simulink model "untitled"  (R2021a)
settings: Solver=VariableStepAuto  StartTime=0.0  StopTime=10.0  RelTol=1e-3
settings Model: Creator=nguye  LastModifiedBy=nguye

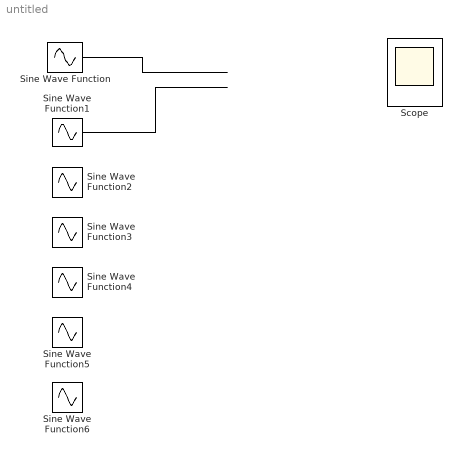
== system untitled ==
  Scope : Scope
  Sine Wave Function : Sin  Amplitude=2  Frequency=30  Phase=pi/2  SampleTime=1/10000
  Sine Wave Function1 : Sin  Amplitude=0.08  Frequency=30  Phase=0.05*pi  SampleTime=1/10000
  Sine Wave Function{2..6} (5 alike) : Sin  TimeSource=Use external signal  SampleTime=0
  wires:
  Sine Wave Function/1 -> ?
  Sine Wave Function1/1 -> ?
  ? -> Scope/1
